simulink model "uselessModel"  (R2019b)
settings: Solver=VariableStepAuto  StartTime=0.0  StopTime=10.0  RelTol=1e-3
settings Model: Creator=sidha  LastModifiedBy=sidha

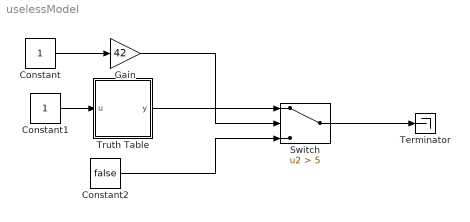
== system uselessModel ==
  Constant : Constant
  Constant1 : Constant
  Constant2 : Constant  Value=false
  Gain : Gain  Gain=42
  Switch : Switch  Criteria=u2 > Threshold  Threshold=5
  Terminator : Terminator
  Truth Table : Truth Table  TreatAsAtomicUnit=on
  wires:
  Constant/1 -> Gain/1
  Constant1/1 -> Truth Table/1(u)
  Truth Table/1(y) -> Switch/1
  Constant2/1 -> Switch/3
  Gain/1 -> Switch/2
  Switch/1 -> Terminator/1

== matlab function uselessModel/Truth Table ==
  data: u input; y output
function y = fcn(u)

aVarTruthTableCondition_1 = false;
aVarTruthTableCondition_2 = false;


% Example condition 1

aVarTruthTableCondition_1 = logical(u >= 0);

% Example condition 2

aVarTruthTableCondition_2 = logical(u ^ 2 <= 1);

if (aVarTruthTableCondition_1 && aVarTruthTableCondition_2)
    aFcnTruthTableAction_1();
elseif (~aVarTruthTableCondition_1 && ~aVarTruthTableCondition_2)
    aFcnTruthTableAction_1();
else % Default
    aFcnTruthTableAction_2();
end

function aFcnTruthTableAction_1()

% Example action 1 called from D1 & D2 column in condition table

y = u;

function aFcnTruthTableAction_2()

% Example action 2 called from D3 column in condition table

y = 1 / u;
